simulink model "Chinhtungservo_theovitri"  (R2016a)
settings: Solver=FixedStepDiscrete  StartTime=0.0  StopTime=inf  FixedStep=0.02  RelTol=1e-3
InitFcn:
  | ts = 0.02;
values from neighbouring files (symbols this model uses):
  deta = [0 0.00107213393654 0.00416893050117 0.00911083471691 0.0157178622249 0.0238092902406 0.0332034061222 0.0437173795929 0.0551672976295 0.0673683764533 0.080135343036 0.0932829594985 ... (1212 elements, 101x12)]    [dang1.mat]    (also in dang3.mat = [0 0.00112687810751 0.00436390592225 0.00949550865103 0.0163; dang4.mat = [0 0.00183366934445 0.00704247991907 0.015187473155 0.025827)
libraries: arduinolib x1
settings Model: SimulationMode=external  ExtModeTrigDuration=2  Creator=Khuu Bach Thy  LastModifiedBy=ACER
settings OptimizationCC: OptimizeModelRefInitCode=on  LifeSpan=Inf  MaxStackSize=64
settings HardwareCC: ProdBitPerPointer=32  ProdLargestAtomicInteger=Long  ProdLargestAtomicFloat=Double  ProdWordSize=32  ProdHWDeviceType=ARM Compatible->ARM Cortex
settings RTWCC: SystemTargetFile=ert.tlc  HardwareBoard=Arduino Due  TemplateMakefile=ert_default_tmf  GenerateReport=on  Toolchain=Arduino ARM v1.6.1  BuildConfiguration=Faster Runs  IncludeHyperlinkInReport=on  LaunchReport=on  GenerateTraceInfo=on  GenerateTraceReport=on  GenerateTraceReportSl=on  GenerateTraceReportSf=on  GenerateTraceReportEml=on
settings CodeAppCC: ForceParamTrailComments=on  IgnoreCustomStorageClasses=off  OperatorAnnotations=on  SimulinkDataObjDesc=on  SFDataObjDesc=on  MATLABFcnDesc=on  InsertBlockDesc=on  MATLABSourceComments=on
settings ERTTargetCC: SupportContinuousTime=on  SupportVariableSizeSignals=on

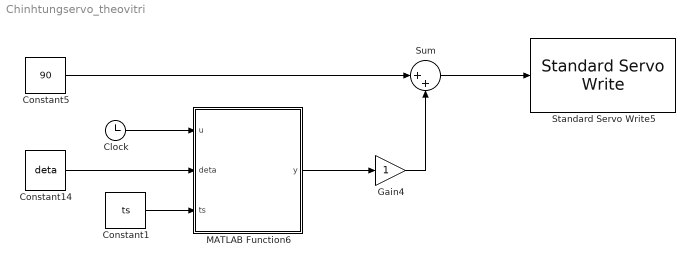
== system Chinhtungservo_theovitri ==
  Clock : Clock
  Constant1 : Constant  Value=ts  SampleTime=0.02
  Constant14 : Constant  Value=deta
  Constant5 : Constant  Value=90  SampleTime=0.02
  Gain4 : Gain
  MATLAB Function6 : MATLAB Function  TreatAsAtomicUnit=on
  Standard Servo Write5 : arduinolib/Standard Servo Write  pinNumber=2  blockPlatform=arduino
  Sum : Sum  Inputs=|++
  wires:
  Sum/1 -> Standard Servo Write5/1
  Constant5/1 -> Sum/1
  Gain4/1 -> Sum/2
  MATLAB Function6/1(y) -> Gain4/1
  Constant14/1 -> MATLAB Function6/2(deta)
  Constant1/1 -> MATLAB Function6/3(ts)
  Clock/1 -> MATLAB Function6/1(u)

== matlab function Chinhtungservo_theovitri/MATLAB Function6 ==
  data: u input; y output; deta input; ts input
function y = fcn(u,deta,ts)
%#codegen

deta2=deta(: , 1);
Deta2=deta2*180/pi;
k = mod(round(u/ts), 101)+1;

y=Deta2(k);
